simulink model "blankpage"  (R2018a)
settings: Solver=ode4  StartTime=0.0  StopTime=endTime  FixedStep=timeStep  RelTol=1e-3
model workspace (MAT data in the model file):
  endTime = 12
  propulsion.pvessel.temperatureBreakpoints = [-90.82 -90 -88.46 -85 -80 -75 -70 -65 -60 -55 -50 -45 -40 -35 -30 -25 -20 -15 -10 -5 0 5 10 15 20 25 30 35 36.42]
  propulsion.pvessel.pressure = [87.73 92.29 101.325 124.2 164.2 213.6 273.6 345.7 431.5 532.3 649.9 785.8 941.7 1119 1321 1547 1801 2083 2397 2744 3127 3547 4007 4510 5060 5660 6315 7033 7251]
  propulsion.pvessel.initOxiMass = 11.3959561341
  propulsion.pvessel.initVapMass = 0.910928351853
  propulsion.pvessel.initLiqMass = 10.4850277822
  propulsion.pvessel.initOxiTemp = 30
  propulsion.pvessel.liqDensity = [1222.8 1220.6 1216.3 1206.7 1192.7 1178.3 1163.7 1148.8 1133.6 1118 1118 1085.6 1068.8 1051.4 1033.4 1014.8 995.4 975.2 953.9 931.4 907.4 881.6 853.5 822.2 786.6 743.9 688 589.4 452]
  propulsion.pvessel.vapDensity = [2.613 2.738 2.987 3.609 4.68 5.982 7.546 9.406 11.6 14.16 17.14 20.58 24.53 29.05 34.22 40.11 46.82 54.47 63.21 73.26 84.86 98.41 114.5 133.9 158.1 190 236.7 330.4 452]
  propulsion.pvessel.delHVap = [377 377 375 371 365 359 353 346 340 333 326 318 310 302 294 285 276 266 255 244 232 219 204 188 169 147 117 64.9 0]
  propulsion.pvessel.specHeatCap = [1.747 1.75 1.756 1.768 1.781 1.791 1.798 1.803 1.807 1.812 1.818 1.827 1.84 1.858 1.833 1.915 1.957 2.011 2.079 2.166 2.274 2.412 2.592 2.834 3.188 3.781 5.143 10 100]
  propulsion.pvessel.lengthVP = 0.25
  propulsion.pvessel.n2o_pCrit = 7251
  propulsion.pvessel.n2o_rhoCrit = 452
  propulsion.pvessel.n2o_tCrit = 36.42
  propulsion.pvessel.n2o_ZCrit = 0.28
  propulsion.pvessel.n2o_gamma = 1.3
  propulsion.pvessel.L_OxiTank = 1.24
  propulsion.pvessel.D_OxiTank = 0.14
  propulsion.pvessel.volumeTank = 0.0190883169632
  propulsion.pvessel.name = 'pvessel'
  propulsion.pvessel.libraryLoc = 'elementsLibrary/pvessel'
  propulsion.pvessel.initialized = 1
  propulsion.pvessel.blockChoice = 'nitrousTank1'
  propulsion.pvessel.timeStep = 0.001
  propulsion.A_ih = 2.4476e-06
  propulsion.nIHoles = 16
  propulsion.injector_Cd = 0.45
  propulsion.a = 0.155
  propulsion.n = 0.555
  propulsion.At = 0.001
  propulsion.Ai = 0.001
  propulsion.k = 1.27
  propulsion.gasConst = 385
  propulsion.etaCombustion = 0.95
  propulsion.etaNozzle = 0.98
  propulsion.Dfg_inner = 0.04
  propulsion.Dfg_outer = 0.134
  propulsion.Lfg = 0.3
  propulsion.rho_fuel = 930
  propulsion.initMassFuel = 1.140831
  propulsion.X_GM = 2.244
  propulsion.X_CG_full = 0.2745
  propulsion.Ae = 0.0058
  propulsion.m_wet = 6.258
  propulsion.m_dry = 2.835
  propulsion.name = 'propulsion'
  propulsion.libraryLoc = 'elementsLibrary/propulsion'
  propulsion.initialized = 1
  propulsion.blockChoice = 'HREV1'
  propulsion.timeStep = 0.001
  simInput.time = [0 0.001 0.002 0.003 0.004 0.005 0.006 0.007 0.008 0.009 0.01 0.011 ... (12001 elements, 1x12001)]
  simInput.valveCmd = [0 0 0 0 0 0 0 0 0 0 0 0 ... (12001 elements, 1x12001)]
  simInput.temp_atm = [25 25 25 25 25 25 25 25 25 25 25 25 ... (12001 elements, 1x12001)]
  simInput.pressure_atm = [101.3 101.3 101.3 101.3 101.3 101.3 101.3 101.3 101.3 101.3 101.3 101.3 ... (12001 elements, 1x12001)]
  simInput.density_atm = [1.225 1.225 1.225 1.225 1.225 1.225 1.225 1.225 1.225 1.225 1.225 1.225 ... (12001 elements, 1x12001)]
  timeProfile = [0 0.001 0.002 0.003 0.004 0.005 0.006 0.007 0.008 0.009 0.01 0.011 ... (12001 elements, 1x12001)]
  timeStep = 0.001
libraries: elementsLibrary x1
(part 1 of 2)
settings Model: Creator=Manit  LastModifiedBy=ginoy
settings DataIOCC: SaveOutput=off  DSMLogging=off

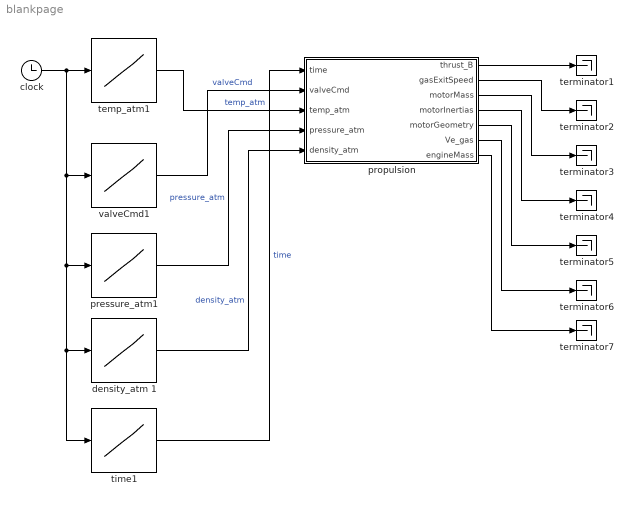
== system blankpage ==
  clock : Clock
  density_atm 1 : Lookup_n-D  NumberOfTableDimensions=1  BreakpointsForDimension1=timeProfile  Table=simInput.density_atm  InternalRulePriority=Speed  RndMeth=Simplest  InputSameDT=on
  pressure_atm1 : Lookup_n-D  NumberOfTableDimensions=1  BreakpointsForDimension1=timeProfile  Table=simInput.pressure_atm  InternalRulePriority=Speed  RndMeth=Simplest  InputSameDT=on
  propulsion : Subsystem  BlockChoice=HREV1
      settings: AttributesFormatString=%<BlockChoice>  TemplateBlock=elementsLibrary/propulsion  MemberBlocks=HREV1,SolidMotor
  temp_atm1 : Lookup_n-D  NumberOfTableDimensions=1  BreakpointsForDimension1=timeProfile  Table=simInput.temp_atm  InternalRulePriority=Speed  RndMeth=Simplest  InputSameDT=on
  terminator{1..7} (7 alike) : Terminator
  time1 : Lookup_n-D  NumberOfTableDimensions=1  BreakpointsForDimension1=timeProfile  Table=simInput.time  InternalRulePriority=Speed  RndMeth=Simplest  InputSameDT=on
  valveCmd1 : Lookup_n-D  NumberOfTableDimensions=1  BreakpointsForDimension1=timeProfile  Table=simInput.valveCmd  InternalRulePriority=Speed  RndMeth=Simplest  InputSameDT=on
  wires:
  clock/1 -> time1/1, density_atm 1/1, pressure_atm1/1, valveCmd1/1, temp_atm1/1
  propulsion/7(engineMass) -> terminator7/1
  propulsion/6(Ve_gas) -> terminator6/1
  propulsion/5(motorGeometry) -> terminator5/1
  propulsion/4(motorInertias) -> terminator4/1
  propulsion/3(motorMass) -> terminator3/1
  propulsion/2(gasExitSpeed) -> terminator2/1
  propulsion/1(thrust_B) -> terminator1/1
  density_atm 1/1 -> propulsion/5("density_atm ")  "density_atm"
  pressure_atm1/1 -> propulsion/4(pressure_atm)  "pressure_atm"
  temp_atm1/1 -> propulsion/3(temp_atm)  "temp_atm"
  valveCmd1/1 -> propulsion/2(valveCmd)  "valveCmd"
  time1/1 -> propulsion/1(time)  "time"
